simulink model "main_Sfn_1_2020"  (R2020b)
settings: Solver=FixedStepDiscrete  StartTime=0.0  StopTime=10.0  FixedStep=1  RelTol=1e-3
libraries: sldvlib x16, simulink x1
settings Model: Creator=ayj  LastModifiedBy=adije
settings OptimizationCC: DefaultParameterBehavior=Inlined  UseDivisionForNetSlopeComputation=on  GainParamInheritBuiltInType=on  UseFloatMulNetSlope=on  InlineInvariantSignals=on  PassReuseOutputArgsAs=Individual arguments  ZeroExternalMemoryAtStartup=off  ZeroInternalMemoryAtStartup=off  NoFixptDivByZeroProtection=on  EfficientFloat2IntCast=on  LifeSpan=1  OptimizeBlockOrder=speed  DifferentSizesBufferReuse=on  EfficientTunableParamExpr=on
settings DebuggingCC: ParameterTunabilityLossMsg=error  UnconnectedInputMsg=none  UnconnectedOutputMsg=none  UnconnectedLineMsg=none  SFMachineParentedDataDiag=error
settings HardwareCC: ProdLongLongMode=on
settings SFSimCC: MATLABDynamicMemAlloc=off
settings RTWCC: Description=Embedded Coder  SystemTargetFile=ert.tlc  TemplateMakefile=ert_default_tmf
settings CodeAppCC: ForceParamTrailComments=on  IgnoreCustomStorageClasses=off  OperatorAnnotations=on  SimulinkDataObjDesc=on  SFDataObjDesc=on  CustomSymbolStrGlobalVar=rt$N$M  CustomSymbolStrType=$N$M  CustomSymbolStrFcn=$N$M$F  CustomSymbolStrMacro=$N$M  InsertBlockDesc=on
settings ERTTargetCC: TargetLangStandard=C99 (ISO)  GenerateSampleERTMain=on  IncludeMdlTerminateFcn=off  CombineSignalStateStructs=on  SupportComplex=off  SupportNonInlinedSFcns=on  InlinedParameterPlacement=NonHierarchical  ERTCustomFileTemplate=example_file_process.tlc  ERTFilePackagingFormat=CompactWithDataFile
settings ConfigComp: DVMode=PropertyProving  DVTestSuiteOptimization=Auto  DVDetectOutOfBounds=on  DVProvingStrategy=FindViolation  DVMaxViolationSteps=12

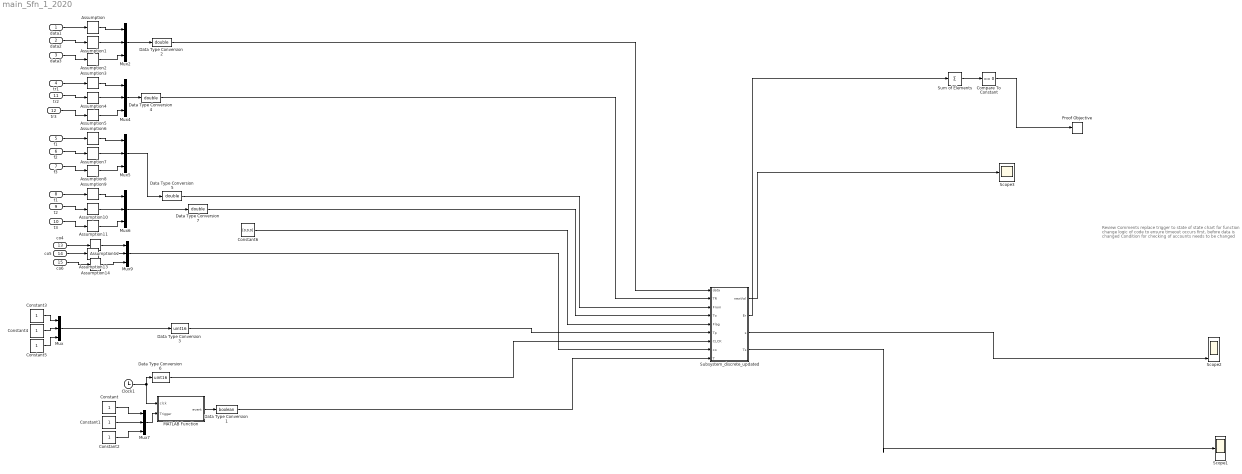
== system main_Sfn_1_2020 ==
  note: Review Comments
      | replace trigger to state of state chart for function
      | change logic of code to ensure timeout occurs first, before data is changed
      | Condition for checking of accounts needs to be changed
  data1 : Inport  OutDataTypeStr=uint16
  data2 : Inport  Port=2  OutDataTypeStr=uint16
  data3 : Inport  Port=3  OutDataTypeStr=uint16
  tr1 : Inport  Port=4  OutDataTypeStr=double
  f1 : Inport  Port=5  OutDataTypeStr=uint16  LockScale=on
  f2 : Inport  Port=6  OutDataTypeStr=uint16
  f3 : Inport  Port=7  OutDataTypeStr=uint16
  t1 : Inport  Port=8  OutDataTypeStr=uint16
  t2 : Inport  Port=9  OutDataTypeStr=uint16
  t3 : Inport  Port=10  OutDataTypeStr=uint16
  tr2 : Inport  Port=11  OutDataTypeStr=double
  tr3 : Inport  Port=12  OutDataTypeStr=double
  co4 : Inport  Port=13
  co5 : Inport  Port=14
  co6 : Inport  Port=15
  Assumption : sldvlib/Objectives and Constraints/Assumption  enabled=on  customAVTBlockType=Assumption  intervals={30}  initial=off  dispValues=on  outEnabled=on
      settings: AttributesFormatString=%<intervals>  SourceProductBaseCode=SL
  Assumption1 : sldvlib/Objectives and Constraints/Assumption  enabled=on  customAVTBlockType=Assumption  intervals={30, 31}  initial=off  dispValues=on  outEnabled=on
      settings: AttributesFormatString=%<intervals>  SourceProductBaseCode=SL
  Assumption10 : sldvlib/Objectives and Constraints/Assumption  enabled=on  customAVTBlockType=Assumption  intervals={2}  initial=off  dispValues=on  outEnabled=on
      settings: AttributesFormatString=%<intervals>  SourceProductBaseCode=SL
  Assumption11 : sldvlib/Objectives and Constraints/Assumption  enabled=on  customAVTBlockType=Assumption  intervals={2}  initial=off  dispValues=on  outEnabled=on
      settings: AttributesFormatString=%<intervals>  SourceProductBaseCode=SL
  Assumption12 : sldvlib/Objectives and Constraints/Assumption  enabled=on  customAVTBlockType=Assumption  intervals={6}  initial=off  dispValues=on  outEnabled=on
      settings: AttributesFormatString=%<intervals>  SourceProductBaseCode=SL
  Assumption13 : sldvlib/Objectives and Constraints/Assumption  enabled=on  customAVTBlockType=Assumption  intervals={6}  initial=off  dispValues=on  outEnabled=on
      settings: AttributesFormatString=%<intervals>  SourceProductBaseCode=SL
  Assumption14 : sldvlib/Objectives and Constraints/Assumption  enabled=on  customAVTBlockType=Assumption  intervals={6}  initial=off  dispValues=on  outEnabled=on
      settings: AttributesFormatString=%<intervals>  SourceProductBaseCode=SL
  Assumption2 : sldvlib/Objectives and Constraints/Assumption  enabled=on  customAVTBlockType=Assumption  intervals={30}  initial=off  dispValues=on  outEnabled=on
      settings: AttributesFormatString=%<intervals>  SourceProductBaseCode=SL
  Assumption3 : sldvlib/Objectives and Constraints/Assumption  enabled=on  customAVTBlockType=Assumption  intervals={-10,+10}  initial=off  dispValues=on  outEnabled=on
      settings: AttributesFormatString=%<intervals>  SourceProductBaseCode=SL
  Assumption4 : sldvlib/Objectives and Constraints/Assumption  enabled=on  customAVTBlockType=Assumption  intervals={-10,+10}  initial=off  dispValues=on  outEnabled=on
      settings: AttributesFormatString=%<intervals>  SourceProductBaseCode=SL
  Assumption5 : sldvlib/Objectives and Constraints/Assumption  enabled=on  customAVTBlockType=Assumption  intervals={-10,+10}  initial=off  dispValues=on  outEnabled=on
      settings: AttributesFormatString=%<intervals>  SourceProductBaseCode=SL
  Assumption6 : sldvlib/Objectives and Constraints/Assumption  enabled=on  customAVTBlockType=Assumption  intervals={1}  initial=off  dispValues=on  outEnabled=on
      settings: AttributesFormatString=%<intervals>  SourceProductBaseCode=SL
  Assumption7 : sldvlib/Objectives and Constraints/Assumption  enabled=on  customAVTBlockType=Assumption  intervals={1}  initial=off  dispValues=on  outEnabled=on
      settings: AttributesFormatString=%<intervals>  SourceProductBaseCode=SL
  Assumption8 : sldvlib/Objectives and Constraints/Assumption  enabled=on  customAVTBlockType=Assumption  intervals={1}  initial=off  dispValues=on  outEnabled=on
      settings: AttributesFormatString=%<intervals>  SourceProductBaseCode=SL
  Assumption9 : sldvlib/Objectives and Constraints/Assumption  enabled=on  customAVTBlockType=Assumption  intervals={2}  initial=off  dispValues=on  outEnabled=on
      settings: AttributesFormatString=%<intervals>  SourceProductBaseCode=SL
  Clock1 : Clock
  Compare To Constant : simulink/Logic and Bit Operations/Compare To Constant  relop===  const=0  OutDataTypeStr=boolean
  Constant{,1..5} (6 alike) : Constant
  Constant6 : Constant  Value=[0,0,0]
  Data Type Conversion1 : DataTypeConversion  OutDataTypeStr=boolean  RndMeth=Round
  Data Type Conversion{2,4..5,7} (4 alike) : DataTypeConversion  OutDataTypeStr=double  RndMeth=Round
  Data Type Conversion3 : DataTypeConversion  OutDataTypeStr=uint16  RndMeth=Round
  Data Type Conversion6 : DataTypeConversion  OutDataTypeStr=uint16  RndMeth=Round
  MATLAB Function : MATLAB Function  TreatAsAtomicUnit=on
  Mux{,2,4..7,9} (7 alike) : Mux  Inputs=3
  Proof Objective : sldvlib/Objectives and Constraints/Proof Objective  enabled=on  customAVTBlockType=Proof Objective  intervals=true  dispValues=on  outEnabled=off  enableStopSim=off
      settings: AttributesFormatString=%<intervals>  SourceProductBaseCode=SL
  Scope1 : Scope  NumInputPorts=3
  Scope2 : Scope  NumInputPorts=3
  Scope3 : Scope
  Subsystem_discrete_updated : Subsystem
  Sum of Elements : Sum  Inputs=+
  wires:
  Clock1/1 -> Data Type Conversion6/1, MATLAB Function/1(clck)
  Constant/1 -> Mux7/1
  Constant1/1 -> Mux7/2
  Constant2/1 -> Mux7/3
  MATLAB Function/1(event) -> Data Type Conversion1/1
  Mux4/1 -> Data Type Conversion4/1
  Mux2/1 -> Data Type Conversion2/1
  data1/1 -> Assumption/1
  data2/1 -> Assumption1/1
  data3/1 -> Assumption2/1
  Assumption/1 -> Mux2/1
  Assumption1/1 -> Mux2/2
  Assumption2/1 -> Mux2/3
  tr3/1 -> Assumption5/1
  Assumption5/1 -> Mux4/3
  Assumption4/1 -> Mux4/2
  tr2/1 -> Assumption4/1
  tr1/1 -> Assumption3/1
  Assumption3/1 -> Mux4/1
  Assumption6/1 -> Mux5/1
  f1/1 -> Assumption6/1
  f2/1 -> Assumption7/1
  Assumption7/1 -> Mux5/2
  Assumption8/1 -> Mux5/3
  f3/1 -> Assumption8/1
  t3/1 -> Assumption11/1
  Assumption11/1 -> Mux6/3
  Assumption10/1 -> Mux6/2
  t2/1 -> Assumption10/1
  t1/1 -> Assumption9/1
  Assumption9/1 -> Mux6/1
  Mux5/1 -> Data Type Conversion5/1
  Mux6/1 -> Data Type Conversion7/1
  Sum of Elements/1 -> Compare To Constant/1
  Compare To Constant/1 -> Proof Objective/1
  Mux7/1 -> MATLAB Function/2(Trigger)
  Constant3/1 -> Mux/1
  Constant4/1 -> Mux/2
  Constant5/1 -> Mux/3
  co4/1 -> Assumption12/1
  co5/1 -> Assumption13/1
  co6/1 -> Assumption14/1
  Data Type Conversion2/1 -> Subsystem_discrete_updated/1(data)
  Data Type Conversion4/1 -> Subsystem_discrete_updated/2(TR)
  Data Type Conversion5/1 -> Subsystem_discrete_updated/3(From)
  Data Type Conversion7/1 -> Subsystem_discrete_updated/4(To)
  Constant6/1 -> Subsystem_discrete_updated/5(Flag)
  Mux9/1 -> Subsystem_discrete_updated/8(co)
  Mux/1 -> Data Type Conversion3/1
  Data Type Conversion6/1 -> Subsystem_discrete_updated/7(CLCK)
  Data Type Conversion1/1 -> Subsystem_discrete_updated/9(T)
  Subsystem_discrete_updated/1(newVal) -> Scope3/1
  Subsystem_discrete_updated/3(s) -> Scope2/3
  Subsystem_discrete_updated/4(Ts) -> Scope1/2
  Data Type Conversion3/1 -> Subsystem_discrete_updated/6(Tp)
  Subsystem_discrete_updated/2(Er) -> Sum of Elements/1
  Assumption12/1 -> Mux9/1
  Assumption13/1 -> Mux9/2
  Assumption14/1 -> Mux9/3

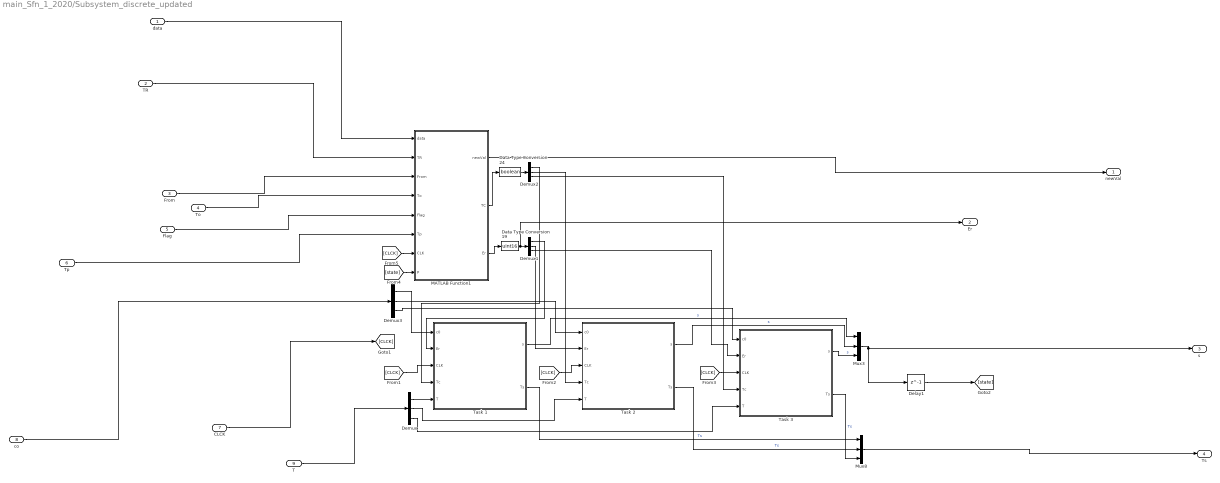
== system main_Sfn_1_2020/Subsystem_discrete_updated ==
  data : Inport
  TR : Inport  Port=2
  From : Inport  Port=3
  To : Inport  Port=4
  Flag : Inport  Port=5
  Tp : Inport  Port=6
  CLCK : Inport  Port=7
  co : Inport  Port=8
  T : Inport  Port=9
  Data Type Conversion19 : DataTypeConversion  OutDataTypeStr=uint16  RndMeth=Round
  Data Type Conversion24 : DataTypeConversion  OutDataTypeStr=boolean  RndMeth=Round
  Delay1 : Delay  DelayLength=1
  Demux{,1..3} (4 alike) : Demux  Outputs=3
  MATLAB Function1 : MATLAB Function  TreatAsAtomicUnit=on
  Mux3 : Mux  Inputs=3
  Mux8 : Mux  Inputs=3
  Task 1 : Stateflow chart  TreatAsAtomicUnit=on
  Task 2 : Stateflow chart  TreatAsAtomicUnit=on
  Task 3 : Stateflow chart  TreatAsAtomicUnit=on
  newVal : Outport
  Er : Outport  Port=2
  s : Outport  Port=3
  Ts : Outport  Port=4
  wires:
  data/1 -> MATLAB Function1/1(data)
  Demux/2 -> Task 2/5(T)
  Demux1/2 -> Task 2/2(Er)
  Mux3/1 -> s/1, Delay1/1
  MATLAB Function1/1(newVal) -> newVal/1
  Demux1/3 -> Task 3/2(Er)
  [CLCK] -> MATLAB Function1/7(CLK)
  Task 2/1(s) -> Mux3/2  "s"
  Mux8/1 -> Ts/1
  Demux3/2 -> Task 2/1(c0)
  [CLCK] -> Task 3/3(CLK)
  Data Type Conversion19/1 -> Er/1, Demux1/1
  Task 1/1(s) -> Mux3/1  "s"
  To/1 -> MATLAB Function1/4(To)
  Demux2/1 -> Task 1/4(Tc)
  [CLCK] -> Task 1/3(CLK)
  Demux2/3 -> Task 3/4(Tc)
  Demux/1 -> Task 1/5(T)
  [CLCK] -> Task 2/3(CLK)
  Flag/1 -> MATLAB Function1/5(Flag)
  Demux3/1 -> Task 1/1(c0)
  Demux3/3 -> Task 3/1(c0)
  Demux2/2 -> Task 2/4(Tc)
  Task 3/2(Ts) -> Mux8/3  "Ts"
  Delay1/1 -> [state]
  Demux/3 -> Task 3/5(T)
  MATLAB Function1/3(Er) -> Data Type Conversion19/1
  MATLAB Function1/2(TC) -> Data Type Conversion24/1
  co/1 -> Demux3/1
  Demux1/1 -> Task 1/2(Er)
  Task 3/1(s) -> Mux3/3  "s"
  Tp/1 -> MATLAB Function1/6(Tp)
  Task 2/2(Ts) -> Mux8/2  "Ts"
  From/1 -> MATLAB Function1/3(From)
  CLCK/1 -> [CLCK]
  Task 1/2(Ts) -> Mux8/1  "Ts"
  [state] -> MATLAB Function1/8(P)
  Data Type Conversion24/1 -> Demux2/1
  T/1 -> Demux/1
  TR/1 -> MATLAB Function1/2(TR)

== stateflow chart main_Sfn_1_2020/Subsystem_discrete_updated/Task 2 ==
  settings: updateMethod=DISCRETE  sampleTime=1
  state Transact
    en:
    s = 1
    Ts = CLK
    du:
    c = c+1
  state Idle
    en:
    c = 0
    s = 0
    Ts = 0
  state Error
    en:
    s = 2
  state Error1
    en:
    s = 3
  Transact -> Error [order 2] : [c>=c0 || Er > 0]
  Idle -> Transact : [T==1]
  (default) -> Idle
  Transact -> Error1 [order 1] : [Tc == 1]
  Error -> Error1
  Error1 -> Idle
  data: c0 input uint16; Er input uint16; CLK input uint16; s output uint16; c local uint16; Ts output uint16; Tc input boolean; T input boolean

== stateflow chart main_Sfn_1_2020/Subsystem_discrete_updated/Task 3 ==
  settings: updateMethod=DISCRETE  sampleTime=1
  state Transact
    en:
    s = 1
    Ts = CLK
    du:
    c = c+1
  state Idle
    en:
    c = 0
    s = 0
    Ts = 0
  state Error
    en:
    s = 2
  state Error1
    en:
    s = 3
  Transact -> Error [order 2] : [c>=c0 || Er > 0]
  Idle -> Transact : [T==1]
  (default) -> Idle
  Transact -> Error1 [order 1] : [Tc == 1]
  Error -> Error1
  Error1 -> Idle
  data: c0 input uint16; Er input uint16; CLK input uint16; s output uint16; c local uint16; Ts output uint16; Tc input boolean; T input boolean

== matlab function main_Sfn_1_2020/MATLAB Function ==
  settings: updateMethod=DISCRETE  sampleTime=1
  data: clck input; event output; Trigger input
function event = fcn(clck, Trigger)
    event = clck==Trigger;

== matlab function main_Sfn_1_2020/Subsystem_discrete_updated/MATLAB Function1 ==
  settings: updateMethod=DISCRETE  sampleTime=1
  data: newVal output; data input double; TR input double; From input double; TC output; To input double; Flag input; Tp input; CLK input; P input; Er output
function [newVal, TC, Er] = fcn(data, TR, From, To, Flag, Tp, CLK, P)
persistent d
persistent f
persistent TC1
persistent Er1
persistent timeo
persistent init
persistent From1
persistent To1
persistent TR1
if(isempty(From1))
    From1 = [1;1;1];
end
if(isempty(To1))
    To1 = [1;1;1];
end
if(isempty(TR1))
    TR1 = [1;1;1];
end
if(isempty(d))
    d = [0;0;0];
end
if(isempty(init))
    init = 0;
end
if(isempty(f))
    f = [0;0;0];
end
if(isempty(TC1))
    TC1 = [0;0;0];
end
if(isempty(Er1))
    Er1 = [0;0;0];
end
if(isempty(timeo))
    timeo = [10,10,10];
end
if(init == 0)
    From1 = From;
    To1 = To;
    TR1 = TR;
    d = data;
    init = 1;
    f = Flag;
end


for i = 1:3
    if P(i) == 1
        if (f(From1(i)) == 0 && f(To1(i)) == 0)
            f(From1(i)) = 1;
            f(To1(i)) = 1;
            timeo(i) = CLK + Tp(i);
            if(d(From1(i)) + TR1(i) < 0 || d(To1(i)) - TR1(i) < 0)
                Er1(i) = 2;
                timeo(i) = 0;
            end
        end
        if CLK >= timeo(i)
            if(Er1(i) ~= 2)
                d(From1(i)) = d(From1(i)) + TR1(i);
                d(To1(i)) = d(To1(i)) - TR1(i);
                TC1(i) = 1;
            end
            f(From1(i)) = 0;
            f(To1(i)) = 0;
        end
    elseif P(i) == 2
        Er1(i) = 1;
    end
end

TC = TC1;
Er = Er1;
newVal = d;

== stateflow chart main_Sfn_1_2020/Subsystem_discrete_updated/Task 1 ==
  settings: updateMethod=DISCRETE  sampleTime=1
  state Transact
    en:
    s = 1
    Ts = CLK
    du:
    c = c+1
  state Idle
    en:
    c = 0
    s = 0
    Ts = 0
  state Error
    en:
    s = 2
  state Error1
    en:
    s = 3
  Transact -> Error [order 2] : [c>=c0 || Er > 0]
  Idle -> Transact : [T==1]
  (default) -> Idle
  Transact -> Error1 [order 1] : [Tc == 1]
  Error -> Error1
  Error1 -> Idle
  data: c0 input uint16; Er input uint16; CLK input uint16; s output uint16; c local uint16; Ts output uint16; Tc input boolean; T input boolean; data local
